simulink model "RadSimulink"  (R2020a)
settings: Solver=VariableStepAuto  StartTime=0.0  StopTime=10.0  RelTol=1e-3
values from neighbouring files (symbols this model uses):
  cz = str2num(get(handles.edit2,'string'))    [GUI.m]
  pz = str2num(get(handles.edit1,'string'))    [GUI.m]
  ti = str2num(get(handles.edit5,'string'))    [GUI.m]
  tp = str2num(get(handles.edit4,'string'))    [GUI.m]
  zl = str2num(get(handles.edit3,'string'))    [GUI.m]
libraries: neural x206, fuzblock x2
(part 3 of 3)

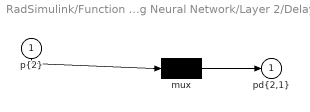
== system RadSimulink/Function Fitting Neural Network/Layer 2/Delays 1 ==
  "p{2}" : Inport  PortDimensions=200
      mask Display: e = 0.06;c1 = [120 230 180]/255;c2 = ([120 230 180]+0)/(256+128);c3 = ([120 230 180]+128)/(256+128);patch([0 1 1 0],[0 0 1 1],c1);patch([0 1 1 1-e 1-e 0+e],[0 0 1 1-e 0+e 0+e],c2);patch([0 0 1 1-e 0+e 0+e],[0 1 1 1-e 1-e 0+e],c3);plot([0 1 1 0 0],[0 0 1 1 0]);
  mux : Mux  Inputs=1
      mask Display: e = 0.06;c1 = [120 150 230]/255;c2 = ([120 150 230]+0)/383;c3 = ([120 150 230]+128)/383;patch([0 1 1 0],[0 0 1 1],c1);patch([0 1 1 1-e 1-e 0+e],[0 0 1 1-e 0+e 0+e],c2);patch([0 0 1 1-e 0+e 0+e],[0 1 1 1-e 1-e 0+e],c3);plot([0 1 1 0 0],[0 0 1 1 0]);disp('Mux')
  "pd{2,1}" : Outport
      mask Display: e = 0.06;c1 = [120 230 180]/255;c2 = ([120 230 180]+0)/(256+128);c3 = ([120 230 180]+128)/(256+128);patch([0 1 1 0],[0 0 1 1],c1);patch([0 1 1 1-e 1-e 0+e],[0 0 1 1-e 0+e 0+e],c2);patch([0 0 1 1-e 0+e 0+e],[0 1 1 1-e 1-e 0+e],c3);plot([0 1 1 0 0],[0 0 1 1 0]);
  wires:
  "p{2}"/1 -> mux/1
  mux/1 -> "pd{2,1}"/1

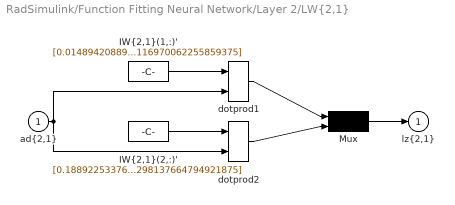
== system RadSimulink/Function Fitting Neural Network/Layer 2/LW{2,1} ==
  "ad{2,1}" : Inport  PortDimensions=200
      mask Display: e = 0.06;c1 = [120 230 180]/255;c2 = ([120 230 180]+0)/(256+128);c3 = ([120 230 180]+128)/(256+128);patch([0 1 1 0],[0 0 1 1],c1);patch([0 1 1 1-e 1-e 0+e],[0 0 1 1-e 0+e 0+e],c2);patch([0 0 1 1-e 0+e 0+e],[0 1 1 1-e 1-e 0+e],c3);plot([0 1 1 0 0],[0 0 1 1 0]);
  "IW{2,1}(1,:)'" : Constant  Value=[0.01489420889954154968159993899234905256889760494232177734375;1.012004217367437508556804459658451378345489501953125;-0.1779140016973787818965746510002645663917064666748046875;0.380890363334270565243144801570451818406581878662109375;-0.045994033123479390046117742940623429603874683380126953125;-0.7994716177916221244714733984437771141529083251953125;0.12073152195305968115146555419414653442800045013427734375;0.8285343366061346248585550711140967905521392822265625;0.9619835750230409932015618323930539190769195556640625;0.76083102905259558657036222939495928585529327392578125;-0.374576263019600286252597243219497613608837127685546875;-0.0324611346768358954850697273286641575396060943603515625;0.94684864696935122641008319988031871616840362548828125;-0.9271715196248582202542820596136152744293212890625;0.28513535260137234939037398362415842711925506591796875;-0.495055291074318670752063553663901984691619873046875;0.7803725950817181900021068940986879169940948486328125;-0.51415989366705916463473613475798629224300384521484375;-0.2051539913855743024750921676968573592603206634521484375;-0.26946546942388105438936918289982713758945465087890625;0.83550967453216318236997040003188885748386383056640625;1.07658762726345091920165941701270639896392822265625;-0.0133439890618509103548117167292730300687253475189208984375;-0.8359102756763994168665021788910962641239166259765625;-0.4448290084054813409153439351939596235752105712890625;0.0961630030102128829927465858418145217001438140869140625;0.047417207448406405168039867703555501066148281097412109375;-0.6277903108022708789093258019420318305492401123046875;-0.485649942980200310937988206205773167312145233154296875;-0.8516174578683621820829330317792482674121856689453125;0.88814414975845623612116241929470561444759368896484375;-0.59620245680741634775046122740604914724826812744140625;-0.47859635814444645429688307558535598218441009521484375;-0.80822948602303112952682795366854406893253326416015625;-0.53429964766247362017992372784647159278392791748046875;-0.59451402015562815339677626980119384825229644775390625;-1.2853851862223615309943625106825493276119232177734375;0.412397489225905189424992158819804899394512176513671875;0.484629435690054288787820269135409034788608551025390625;0.98332487045043770468311095100943930447101593017578125;-0.9555173134025347625453150612884201109409332275390625;-0.42908633323065126230488885994418524205684661865234375;-0.58287942431879058435839624507934786379337310791015625;-1.0081106096434890861957001106929965317249298095703125;-0.310481361560766000451394575065933167934417724609375;0.058363220358028711221010098597616888582706451416015625;0.451738838523741581543191614400711841881275177001953125;-1.387227806171257071810032357461750507354736328125;-0.0204464540201055137991215104875664110295474529266357421875;-0.96907738025416800820011076211812905967235565185546875;-0.15362084468783676616254751934320665895938873291015625;0.78290107174966572234353634485160000622272491455078125;0.322549589560199356785830104854539968073368072509765625;-0.6892347614453433468639786951825954020023345947265625;0.9357254708859426006739568038028664886951446533203125;0.481154804847429840020112123966100625693798065185546875;-1.0553661426129037348431438658735714852809906005859375;0.416422563911451770746197098560514859855175018310546875;0.47148847620154132886938214141991920769214630126953125;-0.36222234068803105255796026540338061749935150146484375;0.1470156067418267598068126744692563079297542572021484375;0.81827085473291638617610033179516904056072235107421875;0.470139511905156404214523035989259369671344757080078125;-0.99510318032028777235353800278971903026103973388671875;-0.5707914563783604844360297647654078900814056396484375;-0.360654334896794936948793974806903861463069915771484375;0.52106154372992496970340425832546316087245941162109375;-1.3403375269110127110394614646793343126773834228515625;-1.1590305686424777764642612964962609112262725830078125;-1.2227657627290910991035843835561536252498626708984375 ...(+7303 chars)]
      mask Display: e = 0.06;c1 = [120 150 230]/255;c2 = ([120 150 230]+0)/383;c3 = ([120 150 230]+128)/383;patch([0 1 1 0],[0 0 1 1],c1);patch([0 1 1 1-e 1-e 0+e],[0 0 1 1-e 0+e 0+e],c2);patch([0 0 1 1-e 0+e 0+e],[0 1 1 1-e 1-e 0+e],c3);plot([0 1 1 0 0],[0 0 1 1 0]);disp('weights');
  "IW{2,1}(2,:)'" : Constant  Value=[0.188922533769830369720921225962229073047637939453125;0.91323815707310485034753355648717842996120452880859375;-0.54271760224595688715254482303862459957599639892578125;-0.7361859307964653265088372791069559752941131591796875;0.86796091937366226520822465317905880510807037353515625;-0.46352202594270097701922850319533608853816986083984375;0.319871926357325586653956861482583917677402496337890625;-0.53623909932731661509563991785398684442043304443359375;-0.10535451794687684945461825236634467728435993194580078125;0.305402489879481542356387535619433037936687469482421875;-0.16737396788772429534475350010325200855731964111328125;0.82718758778630918637730928821838460862636566162109375;-0.819667042889738350908146458095870912075042724609375;0.66670490564060458371642425845493562519550323486328125;-0.94213244267952678256961007718928158283233642578125;0.9717997181606350398652693911571986973285675048828125;-0.77195950125398427044132176888524554669857025146484375;-0.5698223138583260460876545039354823529720306396484375;0.2087392402355659759560779775711125694215297698974609375;0.236531384944102585077274625291465781629085540771484375;-0.9518251392711534197843548099626787006855010986328125;0.260732715326996211668841851860634051263332366943359375;0.88523372030911728902680124519974924623966217041015625;0.16508244041524500200779357328428886830806732177734375;-0.8708702347170831359335352317430078983306884765625;0.68659783485992631479888359535834752023220062255859375;0.585604965510940989048549454309977591037750244140625;0.2247038781389447958947158667797339148819446563720703125;-0.350339139716525360679355571846826933324337005615234375;0.5175781700666133300359206259599886834621429443359375;0.52527547848162381427528089261613786220550537109375;0.7077075634115168600857259662006981670856475830078125;-0.5382505598768574373025330714881420135498046875;0.7338778817148321476082628578296862542629241943359375;0.04806921734092063636101244128440157510340213775634765625;-0.360122785346871088218989598317421041429042816162109375;-0.050567763745527523344680531636186060495674610137939453125;0.389386694259850008048573499763733707368373870849609375;-0.1670535012663772744812007431391975842416286468505859375;-0.335964540403287659220410432681092061102390289306640625;-0.67951103363829667980411386452033184468746185302734375;-1.0622679181520140456740364243160001933574676513671875;0.7506992886474617154846100675058551132678985595703125;0.66503129081657608168143269722349941730499267578125;-0.434469429200937617974176419011200778186321258544921875;0.016198794308470876313066355578484944999217987060546875;-0.56058818233474860814880003090365789830684661865234375;0.357749467191739112248427545637241564691066741943359375;-0.11907933410768332949114522989475517533719539642333984375;0.6116606454875908038815168765722773969173431396484375;-0.7536797814538160888986340069095604121685028076171875;-0.720941283756943551708218365092761814594268798828125;0.0225799360888392745827513152789833839051425457000732421875;0.70829033640644556424348365908372215926647186279296875;0.32477578879481949769569837371818721294403076171875;-0.7394323862974514494084132820717059075832366943359375;-0.280753558346979847915036998529103584587574005126953125;0.30075524448948065536768581296200864017009735107421875;-0.850933276848680808512881412752903997898101806640625;0.0961270595072454547835860694249277003109455108642578125;0.735417399007989303072463371790945529937744140625;0.349843769994277409285388102944125421345233917236328125;0.228889966823421941999328055317164398729801177978515625;0.1732421349158871082263289054026245139539241790771484375;-0.2477049112132929942209358387117390520870685577392578125;-1.2264875295548780531618149325367994606494903564453125;-0.273485692484016051917450340624782256782054901123046875;0.0765386937428183811160664618000737391412258148193359375;-0.052535259801617197050749297204674803651869297027587890625;-0.0787873232321571193015330436537624336779117584228515625 ...(+7291 chars)]
      mask Display: e = 0.06;c1 = [120 150 230]/255;c2 = ([120 150 230]+0)/383;c3 = ([120 150 230]+128)/383;patch([0 1 1 0],[0 0 1 1],c1);patch([0 1 1 1-e 1-e 0+e],[0 0 1 1-e 0+e 0+e],c2);patch([0 0 1 1-e 0+e 0+e],[0 1 1 1-e 1-e 0+e],c3);plot([0 1 1 0 0],[0 0 1 1 0]);disp('weights');
  Mux : Mux  Inputs=2
      mask Display: e = 0.06;c1 = [120 150 230]/255;c2 = ([120 150 230]+0)/383;c3 = ([120 150 230]+128)/383;patch([0 1 1 0],[0 0 1 1],c1);patch([0 1 1 1-e 1-e 0+e],[0 0 1 1-e 0+e 0+e],c2);patch([0 0 1 1-e 0+e 0+e],[0 1 1 1-e 1-e 0+e],c3);plot([0 1 1 0 0],[0 0 1 1 0]);disp('Mux');
  dotprod1 : neural/Weight Functions/dotprod
  dotprod2 : neural/Weight Functions/dotprod
  "lz{2,1}" : Outport
      mask Display: e = 0.06;c1 = [120 230 180]/255;c2 = ([120 230 180]+0)/(256+128);c3 = ([120 230 180]+128)/(256+128);patch([0 1 1 0],[0 0 1 1],c1);patch([0 1 1 1-e 1-e 0+e],[0 0 1 1-e 0+e 0+e],c2);patch([0 0 1 1-e 0+e 0+e],[0 1 1 1-e 1-e 0+e],c3);plot([0 1 1 0 0],[0 0 1 1 0]);
  wires:
  "IW{2,1}(1,:)'"/1 -> dotprod1/1
  "ad{2,1}"/1 -> dotprod1/2, dotprod2/2
  dotprod1/1 -> Mux/1
  "IW{2,1}(2,:)'"/1 -> dotprod2/1
  dotprod2/1 -> Mux/2
  Mux/1 -> "lz{2,1}"/1
